simulink model "autopilot"  (R2016b)
settings: Solver=VariableStepAuto  StartTime=0.0  StopTime=250  RelTol=1e-3
values from neighbouring files (symbols this model uses):
  A = [ -0.322 0.052 0.028 -1.12 0.002 ... (first row only)    [constants_part2.m]
  B = [ 0 0 0 0 10]'    [constants_part2.m]
  C = [0 0 0 1 0 ... (first row only)    [constants_part2.m]
  D = [0 0 0]'    [constants_part2.m]
  d = .1*deg2rad    (= 0.00174532925199)    [constants_part2.m]    (also in prob2e.m = 0.1*deg2rad)
  delta_a_max = 25*deg2rad    (= 0.436332312999)    [constants_part2.m]
  g = 9.81    [constants_part2.m]
  h = 0.01    [constants_part2.m]    (also in kalman_filter.m = model_param_struct.h)
  k_d_phi = (2*zeta_phi*omega_n_phi - a_phi_1) / a_phi_2    [constants_part2.m]
  k_i_chi = omega_n_chi^2*V_g/g    [constants_part2.m]
  k_i_phi = -.1    (= -0.1)    [constants_part2.m]
  k_p_chi = 2*zeta_chi*omega_n_chi*V_g/g    [constants_part2.m]
  k_p_phi = delta_a_max / e_phi_max * sign(a_phi_2)    [constants_part2.m]
  V_g = 637/3.6    (= 176.944444444)    [constants_part2.m]
  var_phi = 2^2    (= 4)    [constants_part2.m]
  var_roll_rate = 0.5^2    (= 0.25)    [constants_part2.m]
  var_yaw_rate = 0.2^2    (= 0.04)    [constants_part2.m]
undefined symbols (not defined in the file or in its folder): feedback_select, integratorlowerbound, integratorupperbound, noise_amplifier
libraries: aerolibconvert2 x7
settings Model: Creator=Alexandra  LastModifiedBy=HenningWard

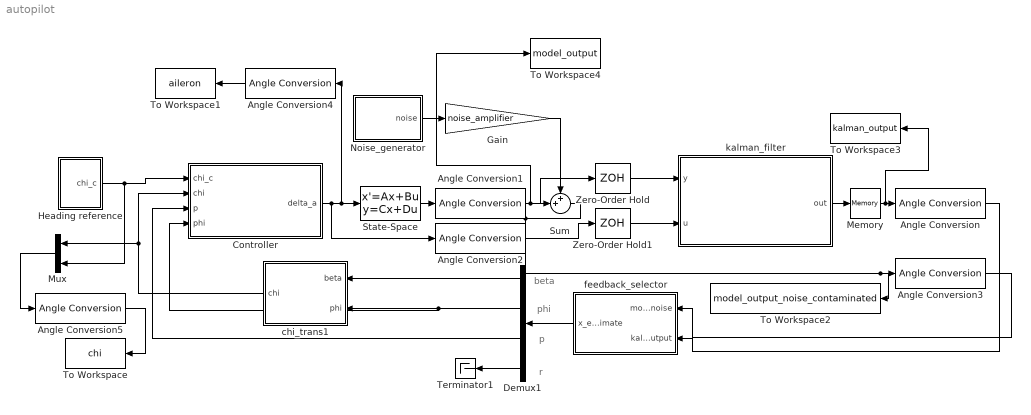
== system autopilot ==
  note: r
  note: p
  note: phi
  note: beta
  Angle Conversion : aerolibconvert2/Angle Conversion  IU=deg  OU=rad
  Angle Conversion{1..2,4..5} (4 alike) : aerolibconvert2/Angle Conversion  IU=rad  OU=deg
  Angle Conversion3 : aerolibconvert2/Angle Conversion  IU=deg  OU=rad
  Controller : Subsystem
  Demux1 : Demux
  Gain : Gain  Gain=noise_amplifier
  Heading reference : Subsystem
  Memory : Memory
  Mux : Mux  Inputs=2
  Noise_generator : Subsystem
  State-Space : StateSpace  A=A  B=B  C=C  D=D  X0=0
  Sum : Sum  Inputs=++|
  Terminator1 : Terminator
  To Workspace : ToWorkspace  VariableName=chi  SaveFormat=Structure With Time  SampleTime=-1
  To Workspace1 : ToWorkspace  VariableName=aileron  SaveFormat=Structure With Time  SampleTime=-1
  To Workspace2 : ToWorkspace  VariableName=model_output_noise_contaminated  SaveFormat=Structure With Time  SampleTime=-1
  To Workspace3 : ToWorkspace  VariableName=kalman_output  SaveFormat=Structure With Time  SampleTime=-1
  To Workspace4 : ToWorkspace  VariableName=model_output  SaveFormat=Structure With Time  SampleTime=-1
  Zero-Order Hold : ZeroOrderHold  SampleTime=h
  Zero-Order Hold1 : ZeroOrderHold  SampleTime=h
  chi_trans1 : Subsystem
  feedback_selector : Subsystem
  kalman_filter : MATLAB Function  TreatAsAtomicUnit=on
  wires:
  Noise_generator/1(noise) -> Gain/1
  Sum/1 -> Zero-Order Hold/1, To Workspace2/1, Angle Conversion3/1
  Zero-Order Hold/1 -> kalman_filter/1(y)
  Controller/1(delta_a) -> Angle Conversion2/1, Angle Conversion4/1, State-Space/1
  kalman_filter/1(out) -> Memory/1
  Heading reference/1("chi_c ") -> Mux/2, Controller/1("chi_c ")
  feedback_selector/1(x_estimate) -> Demux1/1
  Demux1/1 -> chi_trans1/1(beta)
  Demux1/2 -> Controller/4(phi), chi_trans1/2(phi)
  Demux1/3 -> Controller/3(p)
  Demux1/4 -> Terminator1/1
  chi_trans1/1(chi) -> Mux/1, Controller/2("chi ")
  Zero-Order Hold1/1 -> kalman_filter/2(u)
  Memory/1 -> To Workspace3/1, Angle Conversion/1
  Angle Conversion/1 -> feedback_selector/2("kalman_output ")
  State-Space/1 -> Angle Conversion1/1
  Angle Conversion1/1 -> To Workspace4/1, Sum/2
  Angle Conversion2/1 -> Zero-Order Hold1/1
  Angle Conversion3/1 -> feedback_selector/1("model_output w/ noise ")
  Gain/1 -> Sum/1
  Angle Conversion4/1 -> To Workspace1/1
  Angle Conversion5/1 -> To Workspace/1
  Mux/1 -> Angle Conversion5/1

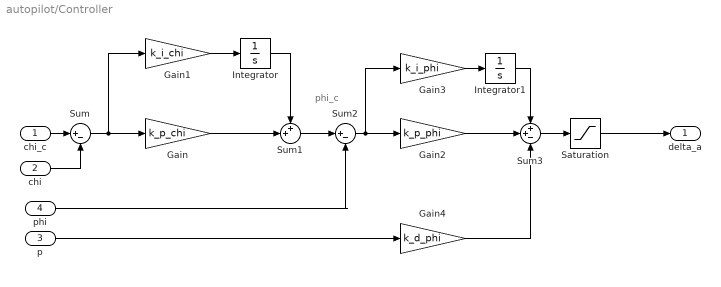
== system autopilot/Controller ==
  note: phi_c
  "chi_c " : Inport
  "chi " : Inport  Port=2
  p : Inport  Port=3
  phi : Inport  Port=4
  Gain : Gain  Gain=k_p_chi
  Gain1 : Gain  Gain=k_i_chi
  Gain2 : Gain  Gain=k_p_phi
  Gain3 : Gain  Gain=k_i_phi
  Gain4 : Gain  Gain=k_d_phi
  Integrator : Integrator  UpperSaturationLimit=integratorupperbound  LowerSaturationLimit=integratorlowerbound
  Integrator1 : Integrator  UpperSaturationLimit=-1  LowerSaturationLimit=integratorlowerbound
  Saturation : Saturate  UpperLimit=delta_a_max  LowerLimit=-delta_a_max
  Sum : Sum  Inputs=|+-
  Sum1 : Sum  Inputs=++|
  Sum2 : Sum  Inputs=|+-
  Sum3 : Sum  Inputs=++-
  delta_a : Outport
  wires:
  p/1 -> Gain4/1
  Saturation/1 -> delta_a/1
  Gain/1 -> Sum1/2
  Sum2/1 -> Gain3/1, Gain2/1
  Sum3/1 -> Saturation/1
  Gain3/1 -> Integrator1/1
  Gain2/1 -> Sum3/2
  Gain4/1 -> Sum3/3
  phi/1 -> Sum2/2
  Sum1/1 -> Sum2/1
  Gain1/1 -> Integrator/1
  Integrator1/1 -> Sum3/1
  Integrator/1 -> Sum1/1
  Sum/1 -> Gain1/1, Gain/1
  "chi_c "/1 -> Sum/1
  "chi "/1 -> Sum/2

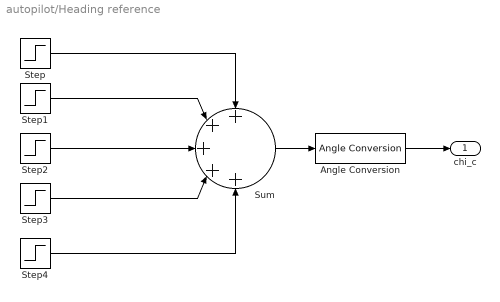
== system autopilot/Heading reference ==
  Angle Conversion : aerolibconvert2/Angle Conversion  IU=deg  OU=rad
  Step : Step  Time=0  After=0  SampleTime=0
  Step1 : Step  Time=50  After=2  SampleTime=0
  Step2 : Step  Time=100  After=4  SampleTime=0
  Step3 : Step  Time=150  After=6  SampleTime=0
  Step4 : Step  Time=200  After=8  SampleTime=0
  Sum : Sum  Inputs=+++++
  "chi_c " : Outport
  wires:
  Step2/1 -> Sum/3
  Step1/1 -> Sum/2
  Step/1 -> Sum/1
  Step3/1 -> Sum/4
  Step4/1 -> Sum/5
  Sum/1 -> Angle Conversion/1
  Angle Conversion/1 -> "chi_c "/1

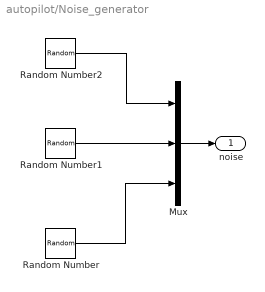
== system autopilot/Noise_generator ==
  Mux : Mux  Inputs=3
  Random Number : RandomNumber  Variance=var_phi  SampleTime=0.1
  Random Number1 : RandomNumber  Variance=var_roll_rate  SampleTime=0.1
  Random Number2 : RandomNumber  Variance=var_yaw_rate  SampleTime=0.1
  noise : Outport
  wires:
  Random Number1/1 -> Mux/2
  Mux/1 -> noise/1
  Random Number2/1 -> Mux/1
  Random Number/1 -> Mux/3

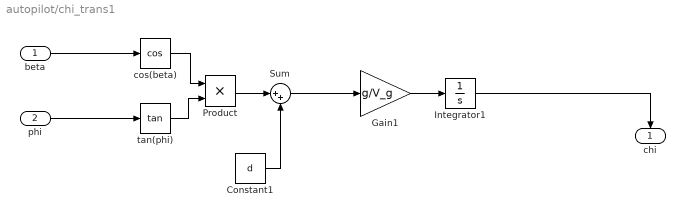
== system autopilot/chi_trans1 ==
  beta : Inport
  phi : Inport  Port=2
  Constant1 : Constant  Value=d
  Gain1 : Gain  Gain=g/V_g
  Integrator1 : Integrator
  Product : Product
  Sum : Sum  Inputs=|++
  cos(beta) : Trigonometry  Operator=cos
  tan(phi) : Trigonometry  Operator=tan
  chi : Outport
  wires:
  phi/1 -> tan(phi)/1
  Integrator1/1 -> chi/1
  beta/1 -> cos(beta)/1
  tan(phi)/1 -> Product/2
  cos(beta)/1 -> Product/1
  Gain1/1 -> Integrator1/1
  Product/1 -> Sum/1
  Sum/1 -> Gain1/1
  Constant1/1 -> Sum/2

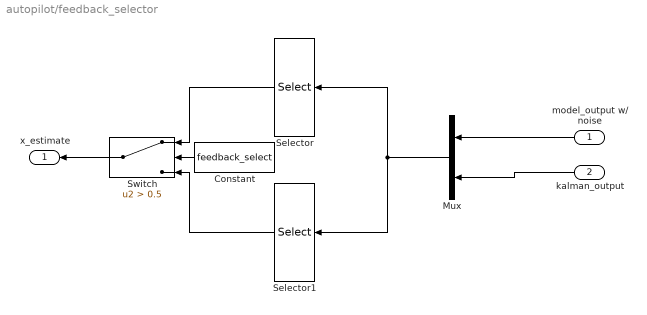
== system autopilot/feedback_selector ==
  "model_output w/ noise " : Inport
  "kalman_output " : Inport  Port=2
  Constant : Constant  Value=feedback_select
  Mux : Mux  Inputs=2
  Selector : Selector  InputPortWidth=7  IndexOptions=Index vector (dialog)  Indices=[4 3 2 1]  OutputSizes=1
  Selector1 : Selector  InputPortWidth=7  IndexOptions=Index vector (dialog)  Indices=[4 5 6 7]  OutputSizes=1
  Switch : Switch  Criteria=u2 > Threshold  Threshold=0.5
  x_estimate : Outport
  wires:
  "kalman_output "/1 -> Mux/2
  "model_output w/ noise "/1 -> Mux/1
  Mux/1 -> Selector/1, Selector1/1
  Selector/1 -> Switch/1
  Selector1/1 -> Switch/3
  Switch/1 -> x_estimate/1
  Constant/1 -> Switch/2

== matlab function autopilot/kalman_filter ==
  data: y input; u input; out output; model_param_struct parameter
function out = kalmanfilter(y, u, model_param_struct)

persistent init_flag x_k P_k;

h   =   model_param_struct.h;

A_d =   model_param_struct.A_d;
B_d =   model_param_struct.B_d;
E_d =   model_param_struct.E_d;
H   =   model_param_struct.C_d;
R   =   model_param_struct.R;
Q   =   model_param_struct.Q;


if isempty(init_flag)
    %initialize enter prior estimate,and error cov;
    init_flag=1;
    x_k = [0;
           0;
           0;
           0];
       
    P_k = eye(4);
    
end

%calculate Kalman gain K_k;
K_k = P_k*H'/(H*P_k*H'+R); 

% update estimate with measured z_k
x_k_ = x_k+K_k*(y-H*x_k);

%compute error covarians
P_k = (eye(4) - K_k*H)*P_k*(eye(4)-K_k*H)'+K_k*R*K_k';

%project ahead
x_k = A_d*x_k_+B_d*u; 
P_k = A_d*P_k*A_d'+E_d*Q*E_d';

out = x_k_;
